simulink model "sw_architecture"  (R2024b)
settings: Solver=VariableStepAuto  StartTime=0.0  StopTime=10.0  RelTol=1e-3
settings Model: Creator=AntonioCaruso  LastModifiedBy=AntonioCaruso

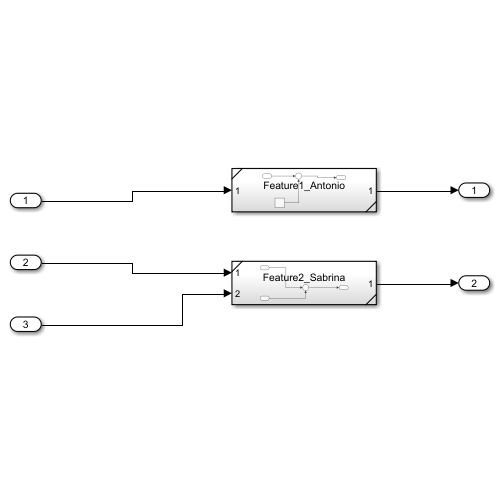
[thumbnail: Simulink's stored preview of the top-level diagram]
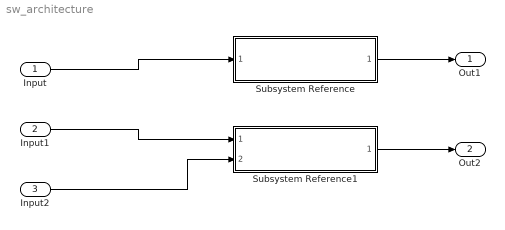
== system sw_architecture ==
  Input : Inport
  Input1 : Inport  Port=2
  Input2 : Inport  Port=3
  Subsystem Reference : Subsystem  ReferencedSubsystem=Feature1_Antonio
  Subsystem Reference1 : Subsystem  ReferencedSubsystem=Feature2_Sabrina
  Out1 : Outport
  Out2 : Outport  Port=2
  wires:
  Input1/1 -> Subsystem Reference1/1
  Input2/1 -> Subsystem Reference1/2
  Input/1 -> Subsystem Reference/1
  Subsystem Reference/1 -> Out1/1
  Subsystem Reference1/1 -> Out2/1
